simulink model "verify_com_acceleration_computation"  (R2015a)
settings: Solver=ode45  StartTime=0.0  StopTime=1.2  RelTol=1e-3
undefined symbols (not defined in the file or in its folder): A_kalman_transverse, A_kalman_vertical, B_kalman_transverse, B_kalman_vertical, C_kalman_transverse, C_kalman_vertical, com_leg_motor, com_torso, Discrete, g, initial_dx_estimate, initial_dy_estimate, initial_dz_estimate, initial_z_estimate, kalman_stance_slip_threshold, lateral_offset, m_leg, m_leg_motor, m_torso, m_total_real, P0_kalman_transverse, P0_kalman_vertical, pelvis_to_imu, R_kalman_accelerometer, R_kalman_foot_slip, R_kalman_foot_stance, sample_time, Time, X, Y, Z
libraries: nesl_utility x121, sm_lib x43, simulink x3, ctrlSharedLib x3
(part 2 of 3)

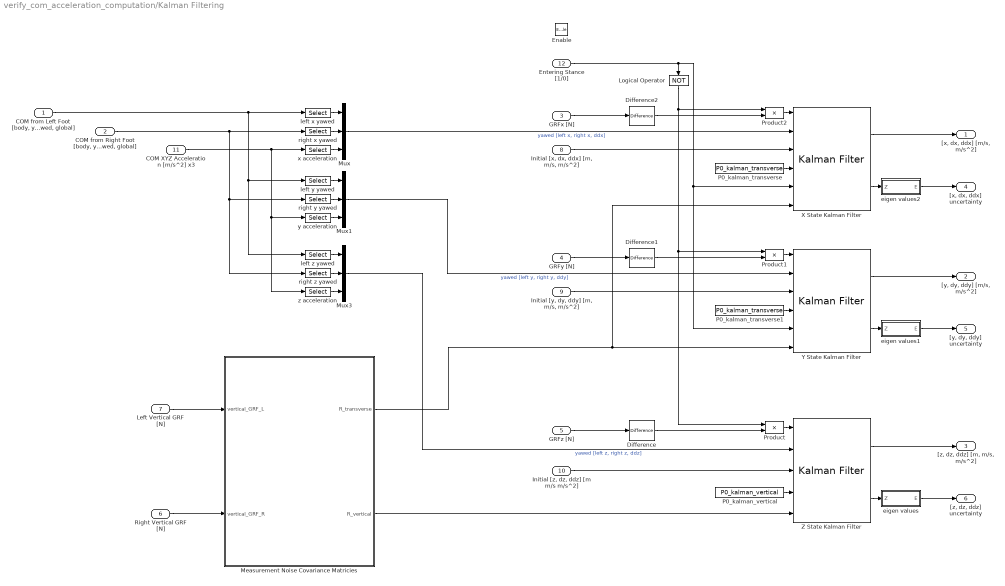
== system verify_com_acceleration_computation/Kalman Filtering ==
  "COM from Left Foot [body, yawed, global]" : Inport  SampleTime=sample_time
  "COM from Right Foot [body, yawed, global]" : Inport  Port=2  SampleTime=sample_time
  GRFx [N] : Inport  Port=3  SampleTime=sample_time
  GRFy [N] : Inport  Port=4  SampleTime=sample_time
  GRFz [N] : Inport  Port=5  SampleTime=sample_time
  Right Vertical GRF [N] : Inport  Port=6  SampleTime=sample_time
  Left Vertical GRF [N] : Inport  Port=7  SampleTime=sample_time
  "Initial [x, dx, ddx] [m, m/s, m/s^2]" : Inport  Port=8  PortDimensions=3  SampleTime=sample_time
  "Initial [y, dy, ddy] [m, m/s, m/s^2]" : Inport  Port=9  PortDimensions=3  SampleTime=sample_time
  "Initial [z, dz, ddz] [m m/s m/s^2]" : Inport  Port=10  PortDimensions=3  SampleTime=sample_time
  COM XYZ Acceleration [m/s^2] x3 : Inport  Port=11  SampleTime=sample_time
  Entering Stance [1/0] : Inport  Port=12  PortDimensions=1  SampleTime=sample_time
  Enable : EnablePort  StatesWhenEnabling=reset
  Difference : simulink/Discrete/Difference  ICPrevInput=0.0  InputProcessing=Inherited  OutMin=[]  OutMax=[]  OutDataType=fixdt(1, 16)  OutScaling=2^-10  DoSatur=off
  Difference1 : simulink/Discrete/Difference  ICPrevInput=0.0  InputProcessing=Inherited  OutMin=[]  OutMax=[]  OutDataType=fixdt(1, 16)  OutScaling=2^-10  DoSatur=off
  Difference2 : simulink/Discrete/Difference  ICPrevInput=0.0  InputProcessing=Inherited  OutMin=[]  OutMax=[]  OutDataType=fixdt(1, 16)  OutScaling=2^-10  DoSatur=off
  Logical Operator : Logic  Operator=NOT  AllPortsSameDT=off  OutDataTypeStr=boolean
  Measurement Noise Covariance Matricies : MATLAB Function  TreatAsAtomicUnit=on
  Mux : Mux  Inputs=3
  Mux1 : Mux  Inputs=3
  Mux3 : Mux  Inputs=3
  P0_kalman_transverse : Constant  Value=P0_kalman_transverse
  P0_kalman_transverse1 : Constant  Value=P0_kalman_transverse
  P0_kalman_vertical : Constant  Value=P0_kalman_vertical
  Product : Product
  Product1 : Product
  Product2 : Product
  X State Kalman Filter : ctrlSharedLib/Kalman Filter  TimeDomain=Discrete-Time  UseCurrentEstimator=on  ModelSource=Individual A, B, C, D matrices  ModelSourceVariable=A_kf  A=A_kalman_transverse  B=B_kalman_transverse  C=C_kalman_transverse  D=0  NumberOfStates=2  NumberOfInputs=1  NumberOfOutputs=2  InitialEstimateSource=Input port  X0=initial_dx_estimate  P0=P0_kalman_transverse  UseK=off  UseGH=on  NumberOfProcessNoiseInputs=1  G=G_kalman_transverse  TimeInvariantG=on  H=0  TimeInvariantH=on  Q=Q_kalman_GRF_difference  TimeInvariantQ=on  R=1  TimeInvariantR=off  N=0  TimeInvariantN=on  AddInputPort=on  AddEnablePort=off  ExternalReset=Rising  OutputEstimatedY=off  OutputP=on  Ts=sample_time
  Y State Kalman Filter : ctrlSharedLib/Kalman Filter  TimeDomain=Discrete-Time  UseCurrentEstimator=on  ModelSource=Individual A, B, C, D matrices  ModelSourceVariable=A_kf  A=A_kalman_transverse  B=B_kalman_transverse  C=C_kalman_transverse  D=0  NumberOfStates=2  NumberOfInputs=1  NumberOfOutputs=2  InitialEstimateSource=Input port  X0=initial_dy_estimate  P0=P0_kalman_transverse  UseK=off  UseGH=on  NumberOfProcessNoiseInputs=1  G=G_kalman_transverse  TimeInvariantG=on  H=0  TimeInvariantH=on  Q=Q_kalman_GRF_difference  TimeInvariantQ=on  R=1  TimeInvariantR=off  N=0  TimeInvariantN=on  AddInputPort=on  AddEnablePort=off  ExternalReset=Rising  OutputEstimatedY=off  OutputP=on  Ts=sample_time
  Z State Kalman Filter : ctrlSharedLib/Kalman Filter  TimeDomain=Discrete-Time  UseCurrentEstimator=on  ModelSource=Individual A, B, C, D matrices  ModelSourceVariable=A_kf  A=A_kalman_vertical  B=B_kalman_vertical  C=C_kalman_vertical  D=0  NumberOfStates=2  NumberOfInputs=1  NumberOfOutputs=2  InitialEstimateSource=Input port  X0=[initial_z_estimate; initial_dz_estimate]  P0=P0_kalman_vertical  UseK=off  UseGH=on  NumberOfProcessNoiseInputs=1  G=G_kalman_vertical  TimeInvariantG=on  H=0  TimeInvariantH=on  Q=Q_kalman_GRF_difference  TimeInvariantQ=on  R=1  TimeInvariantR=off  N=0  TimeInvariantN=on  AddInputPort=on  AddEnablePort=off  OutputEstimatedY=off  OutputP=on  Ts=sample_time
  eigen values : MATLAB Function  TreatAsAtomicUnit=on
  eigen values1 : MATLAB Function  TreatAsAtomicUnit=on
  eigen values2 : MATLAB Function  TreatAsAtomicUnit=on
  left x yawed : Selector  InputPortWidth=9  Indices=[4]
  left y yawed : Selector  InputPortWidth=9  Indices=[5]
  left z yawed : Selector  InputPortWidth=9  Indices=[6]
  right x yawed : Selector  InputPortWidth=9  Indices=[4]
  right y yawed : Selector  InputPortWidth=9  Indices=[5]
  right z yawed : Selector  InputPortWidth=9  Indices=[6]
  x acceleration : Selector  InputPortWidth=3  Indices=[1]
  y acceleration : Selector  InputPortWidth=3  Indices=[2]
  z acceleration : Selector  InputPortWidth=3  Indices=[3]
  "[x, dx, ddx] [m/s, m/s^2]" : Outport
  "[y, dy, ddy] [m/s, m/s^2]" : Outport  Port=2
  "[z, dz, ddz] [m, m/s, m/s^2]" : Outport  Port=3
  "[x, dx, ddx] uncertainty" : Outport  Port=4
  "[y, dy, ddy] uncertainty" : Outport  Port=5
  "[z, dz, ddz] uncertainty" : Outport  Port=6
  wires:
  X State Kalman Filter/1 -> "[x, dx, ddx] [m/s, m/s^2]"/1
  eigen values1/1(E) -> "[y, dy, ddy] uncertainty"/1
  eigen values2/1(E) -> "[x, dx, ddx] uncertainty"/1
  Y State Kalman Filter/1 -> "[y, dy, ddy] [m/s, m/s^2]"/1
  y acceleration/1 -> Mux1/3
  x acceleration/1 -> Mux/3
  z acceleration/1 -> Mux3/3
  COM XYZ Acceleration [m/s^2] x3/1 -> z acceleration/1, y acceleration/1, x acceleration/1
  Z State Kalman Filter/1 -> "[z, dz, ddz] [m, m/s, m/s^2]"/1
  GRFy [N]/1 -> Difference1/1
  Mux3/1 -> Z State Kalman Filter/2  "yawed [left z, right z, ddz]"
  GRFx [N]/1 -> Difference2/1
  Measurement Noise Covariance Matricies/2(R_vertical) -> Z State Kalman Filter/5
  Measurement Noise Covariance Matricies/1(R_transverse) -> X State Kalman Filter/6, Y State Kalman Filter/6
  Mux1/1 -> Y State Kalman Filter/2  "yawed [left y, right y, ddy]"
  Mux/1 -> X State Kalman Filter/2  "yawed [left x, right x, ddx]"
  Right Vertical GRF [N]/1 -> Measurement Noise Covariance Matricies/2(vertical_GRF_R)
  Left Vertical GRF [N]/1 -> Measurement Noise Covariance Matricies/1(vertical_GRF_L)
  "COM from Left Foot [body, yawed, global]"/1 -> left z yawed/1, left y yawed/1, left x yawed/1
  left x yawed/1 -> Mux/1
  "COM from Right Foot [body, yawed, global]"/1 -> right z yawed/1, right y yawed/1, right x yawed/1
  right x yawed/1 -> Mux/2
  left y yawed/1 -> Mux1/1
  right y yawed/1 -> Mux1/2
  left z yawed/1 -> Mux3/1
  right z yawed/1 -> Mux3/2
  P0_kalman_transverse/1 -> X State Kalman Filter/4
  "Initial [x, dx, ddx] [m, m/s, m/s^2]"/1 -> X State Kalman Filter/3
  P0_kalman_transverse1/1 -> Y State Kalman Filter/4
  "Initial [y, dy, ddy] [m, m/s, m/s^2]"/1 -> Y State Kalman Filter/3
  P0_kalman_vertical/1 -> Z State Kalman Filter/4
  "Initial [z, dz, ddz] [m m/s m/s^2]"/1 -> Z State Kalman Filter/3
  X State Kalman Filter/2 -> eigen values2/1(Z)
  Y State Kalman Filter/2 -> eigen values1/1(Z)
  Z State Kalman Filter/2 -> eigen values/1(Z)
  eigen values/1(E) -> "[z, dz, ddz] uncertainty"/1
  Logical Operator/1 -> Product2/1, Product/1, Product1/1
  Difference/1 -> Product/2
  Entering Stance [1/0]/1 -> Y State Kalman Filter/5, X State Kalman Filter/5, Logical Operator/1
  Difference1/1 -> Product1/2
  Difference2/1 -> Product2/2
  Product2/1 -> X State Kalman Filter/1
  Product1/1 -> Y State Kalman Filter/1
  Product/1 -> Z State Kalman Filter/1
  GRFz [N]/1 -> Difference/1

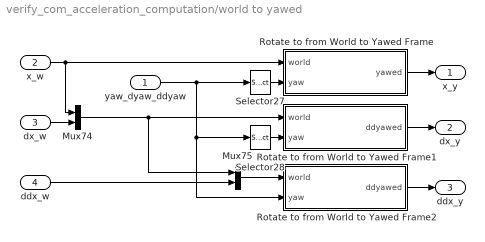
== system verify_com_acceleration_computation/world to yawed ==
  yaw_dyaw_ddyaw : Inport
  x_w : Inport  Port=2
  dx_w : Inport  Port=3
  ddx_w : Inport  Port=4
  Mux74 : Mux  Inputs=2
  Mux75 : Mux  Inputs=2
  Rotate to from World to Yawed Frame : MATLAB Function  TreatAsAtomicUnit=on
  Rotate to from World to Yawed Frame1 : MATLAB Function  TreatAsAtomicUnit=on
  Rotate to from World to Yawed Frame2 : MATLAB Function  TreatAsAtomicUnit=on
  Selector27 : Selector  InputPortWidth=3  Indices=[1]
  Selector28 : Selector  InputPortWidth=3  Indices=[1 2]
  x_y : Outport
  dx_y : Outport  Port=2
  ddx_y : Outport  Port=3
  wires:
  Rotate to from World to Yawed Frame2/1(ddyawed) -> ddx_y/1
  x_w/1 -> Mux74/1, Rotate to from World to Yawed Frame/1(world)
  ddx_w/1 -> Mux75/2
  Mux74/1 -> Mux75/1, Rotate to from World to Yawed Frame1/1(world)
  Mux75/1 -> Rotate to from World to Yawed Frame2/1(world)
  Rotate to from World to Yawed Frame/1(yawed) -> x_y/1
  dx_w/1 -> Mux74/2
  Selector28/1 -> Rotate to from World to Yawed Frame1/2(yaw)
  Rotate to from World to Yawed Frame1/1(ddyawed) -> dx_y/1
  Selector27/1 -> Rotate to from World to Yawed Frame/2(yaw)
  yaw_dyaw_ddyaw/1 -> Selector27/1, Selector28/1, Rotate to from World to Yawed Frame2/2(yaw)

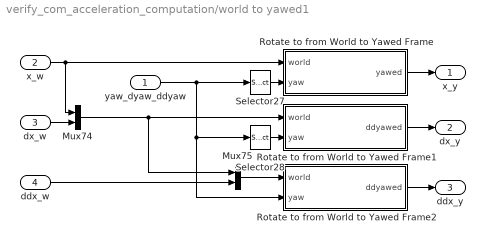
== system verify_com_acceleration_computation/world to yawed1 ==
  yaw_dyaw_ddyaw : Inport
  x_w : Inport  Port=2
  dx_w : Inport  Port=3
  ddx_w : Inport  Port=4
  Mux74 : Mux  Inputs=2
  Mux75 : Mux  Inputs=2
  Rotate to from World to Yawed Frame : MATLAB Function  TreatAsAtomicUnit=on
  Rotate to from World to Yawed Frame1 : MATLAB Function  TreatAsAtomicUnit=on
  Rotate to from World to Yawed Frame2 : MATLAB Function  TreatAsAtomicUnit=on
  Selector27 : Selector  InputPortWidth=3  Indices=[1]
  Selector28 : Selector  InputPortWidth=3  Indices=[1 2]
  x_y : Outport
  dx_y : Outport  Port=2
  ddx_y : Outport  Port=3
  wires:
  Rotate to from World to Yawed Frame2/1(ddyawed) -> ddx_y/1
  x_w/1 -> Mux74/1, Rotate to from World to Yawed Frame/1(world)
  ddx_w/1 -> Mux75/2
  Mux74/1 -> Mux75/1, Rotate to from World to Yawed Frame1/1(world)
  Mux75/1 -> Rotate to from World to Yawed Frame2/1(world)
  Rotate to from World to Yawed Frame/1(yawed) -> x_y/1
  dx_w/1 -> Mux74/2
  Selector28/1 -> Rotate to from World to Yawed Frame1/2(yaw)
  Rotate to from World to Yawed Frame1/1(ddyawed) -> dx_y/1
  Selector27/1 -> Rotate to from World to Yawed Frame/2(yaw)
  yaw_dyaw_ddyaw/1 -> Selector27/1, Selector28/1, Rotate to from World to Yawed Frame2/2(yaw)

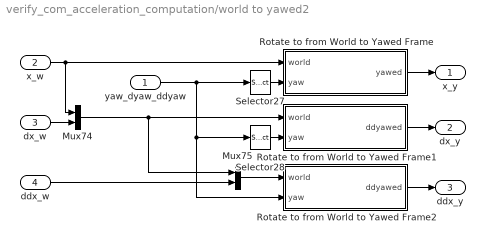
== system verify_com_acceleration_computation/world to yawed2 ==
  yaw_dyaw_ddyaw : Inport
  x_w : Inport  Port=2
  dx_w : Inport  Port=3
  ddx_w : Inport  Port=4
  Mux74 : Mux  Inputs=2
  Mux75 : Mux  Inputs=2
  Rotate to from World to Yawed Frame : MATLAB Function  TreatAsAtomicUnit=on
  Rotate to from World to Yawed Frame1 : MATLAB Function  TreatAsAtomicUnit=on
  Rotate to from World to Yawed Frame2 : MATLAB Function  TreatAsAtomicUnit=on
  Selector27 : Selector  InputPortWidth=3  Indices=[1]
  Selector28 : Selector  InputPortWidth=3  Indices=[1 2]
  x_y : Outport
  dx_y : Outport  Port=2
  ddx_y : Outport  Port=3
  wires:
  Rotate to from World to Yawed Frame2/1(ddyawed) -> ddx_y/1
  x_w/1 -> Mux74/1, Rotate to from World to Yawed Frame/1(world)
  ddx_w/1 -> Mux75/2
  Mux74/1 -> Mux75/1, Rotate to from World to Yawed Frame1/1(world)
  Mux75/1 -> Rotate to from World to Yawed Frame2/1(world)
  Rotate to from World to Yawed Frame/1(yawed) -> x_y/1
  dx_w/1 -> Mux74/2
  Selector28/1 -> Rotate to from World to Yawed Frame1/2(yaw)
  Rotate to from World to Yawed Frame1/1(ddyawed) -> dx_y/1
  Selector27/1 -> Rotate to from World to Yawed Frame/2(yaw)
  yaw_dyaw_ddyaw/1 -> Selector27/1, Selector28/1, Rotate to from World to Yawed Frame2/2(yaw)

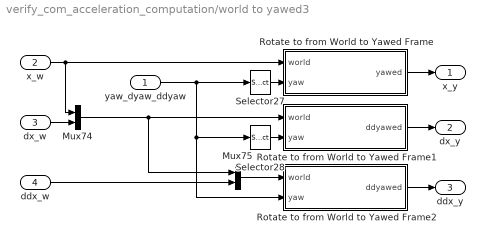
== system verify_com_acceleration_computation/world to yawed3 ==
  yaw_dyaw_ddyaw : Inport
  x_w : Inport  Port=2
  dx_w : Inport  Port=3
  ddx_w : Inport  Port=4
  Mux74 : Mux  Inputs=2
  Mux75 : Mux  Inputs=2
  Rotate to from World to Yawed Frame : MATLAB Function  TreatAsAtomicUnit=on
  Rotate to from World to Yawed Frame1 : MATLAB Function  TreatAsAtomicUnit=on
  Rotate to from World to Yawed Frame2 : MATLAB Function  TreatAsAtomicUnit=on
  Selector27 : Selector  InputPortWidth=3  Indices=[1]
  Selector28 : Selector  InputPortWidth=3  Indices=[1 2]
  x_y : Outport
  dx_y : Outport  Port=2
  ddx_y : Outport  Port=3
  wires:
  Rotate to from World to Yawed Frame2/1(ddyawed) -> ddx_y/1
  x_w/1 -> Mux74/1, Rotate to from World to Yawed Frame/1(world)
  ddx_w/1 -> Mux75/2
  Mux74/1 -> Mux75/1, Rotate to from World to Yawed Frame1/1(world)
  Mux75/1 -> Rotate to from World to Yawed Frame2/1(world)
  Rotate to from World to Yawed Frame/1(yawed) -> x_y/1
  dx_w/1 -> Mux74/2
  Selector28/1 -> Rotate to from World to Yawed Frame1/2(yaw)
  Rotate to from World to Yawed Frame1/1(ddyawed) -> dx_y/1
  Selector27/1 -> Rotate to from World to Yawed Frame/2(yaw)
  yaw_dyaw_ddyaw/1 -> Selector27/1, Selector28/1, Rotate to from World to Yawed Frame2/2(yaw)

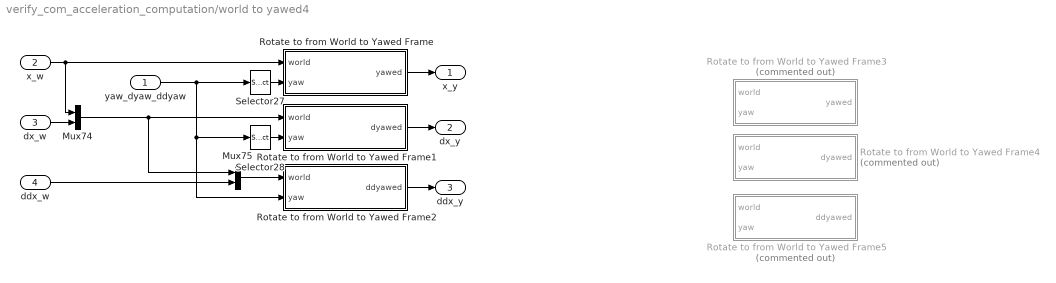
== system verify_com_acceleration_computation/world to yawed4 ==
  yaw_dyaw_ddyaw : Inport
  x_w : Inport  Port=2
  dx_w : Inport  Port=3
  ddx_w : Inport  Port=4
  Mux74 : Mux  Inputs=2
  Mux75 : Mux  Inputs=2
  Rotate to from World to Yawed Frame : MATLAB Function  TreatAsAtomicUnit=on
  Rotate to from World to Yawed Frame1 : MATLAB Function  TreatAsAtomicUnit=on
  Rotate to from World to Yawed Frame2 : MATLAB Function  TreatAsAtomicUnit=on
  Rotate to from World to Yawed Frame3 : MATLAB Function  Commented=on  TreatAsAtomicUnit=on
  Rotate to from World to Yawed Frame4 : MATLAB Function  Commented=on  TreatAsAtomicUnit=on
  Rotate to from World to Yawed Frame5 : MATLAB Function  Commented=on  TreatAsAtomicUnit=on
  Selector27 : Selector  InputPortWidth=3  Indices=[1]
  Selector28 : Selector  InputPortWidth=3  Indices=[1 2]
  x_y : Outport
  dx_y : Outport  Port=2
  ddx_y : Outport  Port=3
  wires:
  yaw_dyaw_ddyaw/1 -> Rotate to from World to Yawed Frame2/2(yaw), Selector28/1, Selector27/1
  Selector27/1 -> Rotate to from World to Yawed Frame/2(yaw)
  Rotate to from World to Yawed Frame1/1(dyawed) -> dx_y/1
  Selector28/1 -> Rotate to from World to Yawed Frame1/2(yaw)
  dx_w/1 -> Mux74/2
  Rotate to from World to Yawed Frame/1(yawed) -> x_y/1
  Mux75/1 -> Rotate to from World to Yawed Frame2/1(world)
  Mux74/1 -> Rotate to from World to Yawed Frame1/1(world), Mux75/1
  ddx_w/1 -> Mux75/2
  x_w/1 -> Rotate to from World to Yawed Frame/1(world), Mux74/1
  Rotate to from World to Yawed Frame2/1(ddyawed) -> ddx_y/1

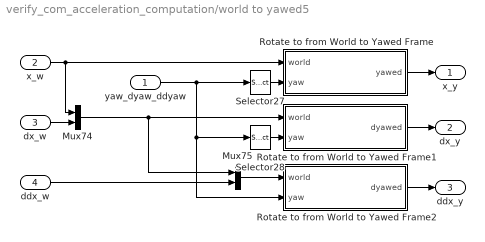
== system verify_com_acceleration_computation/world to yawed5 ==
  yaw_dyaw_ddyaw : Inport
  x_w : Inport  Port=2
  dx_w : Inport  Port=3
  ddx_w : Inport  Port=4
  Mux74 : Mux  Inputs=2
  Mux75 : Mux  Inputs=2
  Rotate to from World to Yawed Frame : MATLAB Function  TreatAsAtomicUnit=on
  Rotate to from World to Yawed Frame1 : MATLAB Function  TreatAsAtomicUnit=on
  Rotate to from World to Yawed Frame2 : MATLAB Function  TreatAsAtomicUnit=on
  Selector27 : Selector  InputPortWidth=3  Indices=[1]
  Selector28 : Selector  InputPortWidth=3  Indices=[1 2]
  x_y : Outport
  dx_y : Outport  Port=2
  ddx_y : Outport  Port=3
  wires:
  Rotate to from World to Yawed Frame2/1(dyawed) -> ddx_y/1
  x_w/1 -> Mux74/1, Rotate to from World to Yawed Frame/1(world)
  ddx_w/1 -> Mux75/2
  Mux74/1 -> Mux75/1, Rotate to from World to Yawed Frame1/1(world)
  Mux75/1 -> Rotate to from World to Yawed Frame2/1(world)
  Rotate to from World to Yawed Frame/1(yawed) -> x_y/1
  dx_w/1 -> Mux74/2
  Selector28/1 -> Rotate to from World to Yawed Frame1/2(yaw)
  Rotate to from World to Yawed Frame1/1(dyawed) -> dx_y/1
  Selector27/1 -> Rotate to from World to Yawed Frame/2(yaw)
  yaw_dyaw_ddyaw/1 -> Selector27/1, Selector28/1, Rotate to from World to Yawed Frame2/2(yaw)

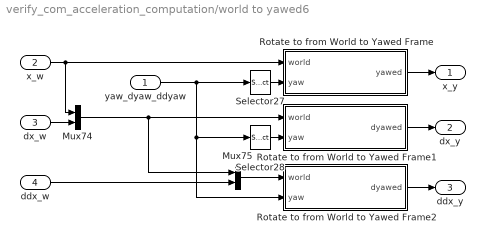
== system verify_com_acceleration_computation/world to yawed6 ==
  yaw_dyaw_ddyaw : Inport
  x_w : Inport  Port=2
  dx_w : Inport  Port=3
  ddx_w : Inport  Port=4
  Mux74 : Mux  Inputs=2
  Mux75 : Mux  Inputs=2
  Rotate to from World to Yawed Frame : MATLAB Function  TreatAsAtomicUnit=on
  Rotate to from World to Yawed Frame1 : MATLAB Function  TreatAsAtomicUnit=on
  Rotate to from World to Yawed Frame2 : MATLAB Function  TreatAsAtomicUnit=on
  Selector27 : Selector  InputPortWidth=3  Indices=[1]
  Selector28 : Selector  InputPortWidth=3  Indices=[1 2]
  x_y : Outport
  dx_y : Outport  Port=2
  ddx_y : Outport  Port=3
  wires:
  yaw_dyaw_ddyaw/1 -> Rotate to from World to Yawed Frame2/2(yaw), Selector28/1, Selector27/1
  Selector27/1 -> Rotate to from World to Yawed Frame/2(yaw)
  Rotate to from World to Yawed Frame1/1(dyawed) -> dx_y/1
  Selector28/1 -> Rotate to from World to Yawed Frame1/2(yaw)
  dx_w/1 -> Mux74/2
  Rotate to from World to Yawed Frame/1(yawed) -> x_y/1
  Mux75/1 -> Rotate to from World to Yawed Frame2/1(world)
  Mux74/1 -> Rotate to from World to Yawed Frame1/1(world), Mux75/1
  ddx_w/1 -> Mux75/2
  x_w/1 -> Rotate to from World to Yawed Frame/1(world), Mux74/1
  Rotate to from World to Yawed Frame2/1(dyawed) -> ddx_y/1

== matlab function verify_com_acceleration_computation/Compute COM Translational Acceleration (IMU uses non-rotating measurement frame) ==
  data: com_acceleration_world output; torso_angular_accelerations input; imu_translational_accelerations_body input; torso_roll input; torso_pitch input; torso_yaw input; com_position_world input; com_velocity_world input; hip_roll_accelerations input; right_hip_roll input; left_hip_roll input; pelvis_to_imu parameter; com_torso parameter; com_leg_motor parameter; m_leg_motor parameter; m_leg parameter; m_torso parameter; torso_com_acceleration_world output; pelvis_acceleration_world output; right_hip_acceleration_world output; left_hip_acceleration_world output; com_acceleration_yawed output
function [com_acceleration_world, torso_com_acceleration_world, pelvis_acceleration_world, right_hip_acceleration_world, left_hip_acceleration_world, com_acceleration_yawed] ...
          = compute_com_acceleration(torso_angular_accelerations, imu_translational_accelerations_body, torso_roll, torso_pitch, torso_yaw, ...
          com_position_world, com_velocity_world, ...
          hip_roll_accelerations, right_hip_roll, left_hip_roll, pelvis_to_imu, com_torso, com_leg_motor, m_leg_motor, m_leg, m_torso)

    % Body frame to Yawed frame rotations  
    R_body_to_yawed = R_pitch(torso_pitch(1))*R_roll(torso_roll(1));
    dR_body_to_yawed = dR_pitch(torso_pitch(1),torso_pitch(2))*R_roll(torso_roll(1)) + R_pitch(torso_pitch(1))*dR_roll(torso_roll(1),torso_roll(2));
    ddR_body_to_yawed = ddR_pitch(torso_pitch(1),torso_pitch(2),torso_angular_accelerations(2))*R_roll(torso_roll(1)) ...
                        + R_pitch(torso_pitch(1))*ddR_roll(torso_roll(1),torso_roll(2),torso_angular_accelerations(1)) ... 
                        + 2*dR_pitch(torso_pitch(1),torso_pitch(2))*dR_roll(torso_roll(1),torso_roll(2));
    % Yawed frame to World frame rotations  
    R_yawed_to_world = R_yaw(torso_yaw(1));
    dR_yawed_to_world = dR_yaw(torso_yaw(1),torso_yaw(2));
    ddR_yawed_to_world = ddR_yaw(torso_yaw(1),torso_yaw(2),torso_angular_accelerations(3));
    % Compute translational acceleration of torso COM
    R_position_body_to_world = R_yawed_to_world*R_body_to_yawed;
    R_velocity_body_to_world = dR_yawed_to_world*R_body_to_yawed + R_yawed_to_world*dR_body_to_yawed;
    R_acceleration_body_to_world = ddR_yawed_to_world*R_body_to_yawed + 2*dR_yawed_to_world*dR_body_to_yawed + R_yawed_to_world*ddR_body_to_yawed;
    imu_to_torso_com_acceleration_world = R_acceleration_body_to_world*(com_torso - pelvis_to_imu)';
    imu_acceleration_world = R_yawed_to_world*R_body_to_yawed*imu_translational_accelerations_body;
    torso_com_acceleration_world = imu_acceleration_world + imu_to_torso_com_acceleration_world;
    % Compute accelerations of hip COMs
    R_right_hip_to_body =     R_roll(-pi/2+right_hip_roll(1));
    dR_right_hip_to_body =   dR_roll(-pi/2+right_hip_roll(1), right_hip_roll(2));
    ddR_right_hip_to_body = ddR_roll(-pi/2+right_hip_roll(1), right_hip_roll(2), hip_roll_accelerations(1));
    R_left_hip_to_body =     R_roll(pi/2-left_hip_roll(1));
    dR_left_hip_to_body =   dR_roll(pi/2-left_hip_roll(1), -left_hip_roll(2));
    ddR_left_hip_to_body = ddR_roll(pi/2-left_hip_roll(1), -left_hip_roll(2), -hip_roll_accelerations(2));
    imu_to_pelvis_com_acceleration_world = R_acceleration_body_to_world*(-pelvis_to_imu)';  
    pelvis_acceleration_world = imu_acceleration_world + imu_to_pelvis_com_acceleration_world;
    left_hip_acceleration_world = pelvis_acceleration_world + (R_acceleration_body_to_world*R_left_hip_to_body + 2*R_velocity_body_to_world*dR_left_hip_to_body + R_position_body_to_world*ddR_left_hip_to_body)*com_leg_motor';
    right_hip_acceleration_world = pelvis_acceleration_world + (R_acceleration_body_to_world*R_right_hip_to_body + 2*R_velocity_body_to_world*dR_right_hip_to_body + R_position_body_to_world*ddR_right_hip_to_body)*(com_leg_motor.*[1,-1,1])';
    % Compute total system COM acceleration
    m_hip = m_leg+m_leg_motor;
    m_total = 2*m_hip + m_torso;
    com_acceleration_world = (m_torso*torso_com_acceleration_world + m_hip*(left_hip_acceleration_world + right_hip_acceleration_world))/m_total;
    com_acceleration_yawed = ddR_yawed_to_world'*com_position_world + 2*dR_yawed_to_world'*com_velocity_world + R_yawed_to_world'*com_acceleration_world;
    %com_acceleration_yawed(3) = com_acceleration_yawed(3) - g;
end

function R_yp = R_pitch(theta) % map from pitched to yawed
  R_yp = [cos(theta), 0, sin(theta); ...
          0, 1, 0; ...
          -sin(theta), 0, cos(theta)];
end
function dR_yp = dR_pitch(theta,dtheta)
  dR_yp = dtheta*[-sin(theta), 0, cos(theta); ...
                  0, 0, 0; ... 
                  -cos(theta), 0, -sin(theta)];
end
function ddR_yp = ddR_pitch(theta,dtheta,ddtheta)
  ddR_yp = ddtheta*[-sin(theta), 0, cos(theta); ...
                    0, 0, 0; ... 
                    -cos(theta), 0, -sin(theta)] ...
           + dtheta^2*[-cos(theta), 0, -sin(theta); ...
                     0, 0, 0; ...
                     sin(theta), 0, -cos(theta)];
end
function R_pr = R_roll(phi) % map from rolled to pitched
  R_pr = [1, 0, 0; ...
          0, cos(phi), -sin(phi); ...
          0, sin(phi), cos(phi)]; 
end
function dR_pr = dR_roll(phi,dphi)
  dR_pr = dphi*[0, 0, 0; ...
                0, -sin(phi), -cos(phi); ...
                0, cos(phi), -sin(phi)];
end
function ddR_pr = ddR_roll(phi, dphi, ddphi)
  ddR_pr = ddphi*[0, 0, 0; ...
                  0, -sin(phi), -cos(phi); ...
                  0, cos(phi), -sin(phi)] ...
           + dphi^2*[0, 0, 0; ...
                   0, -cos(phi), sin(phi);...
                   0, -sin(phi), -cos(phi)];
end
function R_gy = R_yaw(psi) % map yawed frame to global
  R_gy = [cos(psi), -sin(psi), 0; sin(psi), cos(psi), 0; 0 0 1]; 
end
function dR_gy = dR_yaw(psi,dpsi)
  dR_gy = dpsi*[-sin(psi), -cos(psi), 0; cos(psi), -sin(psi), 0; 0 0 0];
end
function ddR_gy = ddR_yaw(psi,dpsi,ddpsi)
  ddR_gy = ddpsi*[-sin(psi), -cos(psi), 0; cos(psi), -sin(psi), 0; 0 0 0] ...
           + dpsi^2*[-cos(psi), sin(psi), 0; -sin(psi), -cos(psi), 0; 0 0 0];
end

== matlab function verify_com_acceleration_computation/Compute COM Translational Acceleration (IMU uses rotating measurement frame)1 ==
  data: com_acceleration_yawed output; torso_angular_accelerations input; imu_translational_positions_body input; imu_translational_velocities_body input; imu_translational_accelerations_body input; torso_roll input; torso_pitch input; hip_roll_accelerations input; right_hip_roll input; left_hip_roll input; pelvis_to_imu parameter; com_torso parameter; com_leg_motor parameter; g parameter; m_leg_motor parameter; m_leg parameter; m_torso parameter; torso_com_acceleration_world output; torso_com_relative_acceleration_world output; torso_com_relative_velocity_world output; imu_to_torso_com_world output; imu_acceleration_world output; imu_velocity_world output; right_hip_acceleration_world output; left_hip_acceleration_world output
function [com_acceleration_yawed,torso_com_acceleration_world,torso_com_relative_acceleration_world,...
          torso_com_relative_velocity_world,imu_to_torso_com_world,imu_acceleration_world,...
          imu_velocity_world, right_hip_acceleration_world, left_hip_acceleration_world] = compute_com_acceleration(torso_angular_accelerations, imu_translational_positions_body, imu_translational_velocities_body, imu_translational_accelerations_body, torso_roll, torso_pitch, hip_roll_accelerations, right_hip_roll, left_hip_roll, pelvis_to_imu, com_torso, com_leg_motor, g, m_leg_motor, m_leg, m_torso)

    % Body frame to Yawed world frame rotations  
    R_body_to_yawed = R_roll(torso_roll(1))*R_pitch(torso_pitch(1));
    dR_body_to_yawed = dR_roll(torso_roll(1),torso_roll(2))*R_pitch(torso_pitch(1)) + R_roll(torso_roll(1))*dR_pitch(torso_pitch(1),torso_pitch(2)); 
    ddR_body_to_yawed = ddR_roll(torso_roll(1),torso_roll(2),torso_angular_accelerations(1))*R_pitch(torso_pitch(1)) ...
                        + R_roll(torso_roll(1))*ddR_pitch(torso_pitch(1),torso_pitch(2),torso_angular_accelerations(2)) ... 
                        + 2*dR_roll(torso_roll(1),torso_roll(2))*dR_pitch(torso_pitch(1),torso_pitch(2)); 
                           
    % Compute translational acceleration of torso COM    
    imu_to_torso_com_world = R_body_to_yawed*(com_torso - pelvis_to_imu)';
    torso_com_relative_velocity_world = dR_body_to_yawed*(com_torso - pelvis_to_imu)';
    torso_com_relative_acceleration_world = ddR_body_to_yawed*(com_torso - pelvis_to_imu)';
    imu_velocity_world = dR_body_to_yawed*imu_translational_positions_body + R_body_to_yawed*imu_translational_velocities_body;
    imu_acceleration_world = ddR_body_to_yawed*imu_translational_positions_body ...
                             + 2*dR_body_to_yawed*imu_translational_velocities_body ...
                             + R_body_to_yawed*imu_translational_accelerations_body;
    torso_com_acceleration_world = imu_acceleration_world + torso_com_relative_acceleration_world;
    
    % Compute accelerations of hip COMs
    R_right_hip_to_body =     R_roll(-pi/2+right_hip_roll(1));
    dR_right_hip_to_body =   dR_roll(-pi/2+right_hip_roll(1), right_hip_roll(2));
    ddR_right_hip_to_body = ddR_roll(-pi/2+right_hip_roll(1), right_hip_roll(2), hip_roll_accelerations(1));
    R_left_hip_to_body =     R_roll(pi/2-left_hip_roll(1));
    dR_left_hip_to_body =   dR_roll(pi/2-left_hip_roll(1), -left_hip_roll(2));
    ddR_left_hip_to_body = ddR_roll(pi/2-left_hip_roll(1), -left_hip_roll(2), -hip_roll_accelerations(2));
    
    pelvis_relative_acceleration_world = ddR_body_to_yawed*(-pelvis_to_imu)';
    pelvis_acceleration_world = imu_acceleration_world + pelvis_relative_acceleration_world;    
    
    left_hip_acceleration_world = pelvis_acceleration_world + (ddR_body_to_yawed*R_left_hip_to_body + 2*(dR_body_to_yawed*dR_left_hip_to_body) + R_body_to_yawed*ddR_left_hip_to_body)*com_leg_motor';
    right_hip_acceleration_world = pelvis_acceleration_world + (ddR_body_to_yawed*R_right_hip_to_body + 2*(dR_body_to_yawed*dR_right_hip_to_body) + R_body_to_yawed*ddR_right_hip_to_body)*(com_leg_motor.*[1,-1,1])';
    
    % Compute total system COM acceleration
    m_hip = m_leg+m_leg_motor;
    m_total = 2*m_hip + m_torso;
    com_acceleration_yawed = (m_torso*torso_com_acceleration_world + m_hip*(left_hip_acceleration_world + right_hip_acceleration_world))/m_total;
     
    
    %com_acceleration_yawed(3) = com_acceleration_yawed(3) - g;
    
end

function R_yp = R_pitch(theta) % map from pitched to yawed
  R_yp = [cos(theta), 0, sin(theta); ...
          0, 1, 0; ...
          -sin(theta), 0, cos(theta)];
end
function dR_yp = dR_pitch(theta,dtheta)
  dR_yp = dtheta*[-sin(theta), 0, cos(theta); ...
                  0, 0, 0; ... 
                  -cos(theta), 0, -sin(theta)];
end
function ddR_yp = ddR_pitch(theta,dtheta,ddtheta)
  ddR_yp = ddtheta*[-sin(theta), 0, cos(theta); ...
                    0, 0, 0; ... 
                    -cos(theta), 0, -sin(theta)] ...
           + dtheta^2*[-cos(theta), 0, -sin(theta); ...
                     0, 0, 0; ...
                     sin(theta), 0, -cos(theta)];
end
function R_pr = R_roll(phi) % map from rolled to pitched
  R_pr = [1, 0, 0; ...
          0, cos(phi), -sin(phi); ...
          0, sin(phi), cos(phi)]; 
end
function dR_pr = dR_roll(phi,dphi)
  dR_pr = dphi*[0, 0, 0; ...
                0, -sin(phi), -cos(phi); ...
                0, cos(phi), -sin(phi)];
end
function ddR_pr = ddR_roll(phi, dphi, ddphi)
  ddR_pr = ddphi*[0, 0, 0; ...
                  0, -sin(phi), -cos(phi); ...
                  0, cos(phi), -sin(phi)] ...
           + dphi^2*[0, 0, 0; ...
                   0, -cos(phi), sin(phi);...
                   0, -sin(phi), -cos(phi)];
end

== matlab function verify_com_acceleration_computation/world to yawed/Rotate to from World to Yawed Frame ==
  data: world input; yawed output; yaw input
function yawed  = WorldToYawed(world, yaw)
    yawed = R_yaw(yaw)'*world;
end

function R_gy = R_yaw(psi) % map yawed frame to global
  R_gy = [cos(psi), -sin(psi), 0; sin(psi), cos(psi), 0; 0 0 1]; 
end

== matlab function verify_com_acceleration_computation/world to yawed/Rotate to from World to Yawed Frame1 ==
  data: world input; ddyawed output; yaw input
function ddyawed  = WorldToYawed(world, yaw)
    ddyawed = dR_yaw(yaw(1),yaw(2))'*world(1:3) + R_yaw(yaw(1))'*world(4:6);
end
function R_gy = R_yaw(psi) % map yawed frame to global
  R_gy = [cos(psi), -sin(psi), 0; sin(psi), cos(psi), 0; 0 0 1]; 
end
function dR_gy = dR_yaw(psi,dpsi)
  dR_gy = dpsi*[-sin(psi), -cos(psi), 0; cos(psi), -sin(psi), 0; 0 0 0];
end

== matlab function verify_com_acceleration_computation/world to yawed/Rotate to from World to Yawed Frame2 ==
  data: world input; ddyawed output; yaw input
function ddyawed  = WorldToYawed(world, yaw)
    ddyawed = ddR_yaw(yaw(1),yaw(2),yaw(3))'*world(1:3) + 2*dR_yaw(yaw(1),yaw(2))'*world(4:6) + R_yaw(yaw(1))'*world(7:9);
end
function R_gy = R_yaw(psi) % map yawed frame to global
  R_gy = [cos(psi), -sin(psi), 0; sin(psi), cos(psi), 0; 0 0 1]; 
end
function dR_gy = dR_yaw(psi,dpsi)
  dR_gy = dpsi*[-sin(psi), -cos(psi), 0; cos(psi), -sin(psi), 0; 0 0 0];
end
function ddR_gy = ddR_yaw(psi,dpsi,ddpsi)
  ddR_gy = ddpsi*[-sin(psi), -cos(psi), 0; cos(psi), -sin(psi), 0; 0 0 0] ...
           + dpsi^2*[-cos(psi), sin(psi), 0; -sin(psi), -cos(psi), 0; 0 0 0];
end

== matlab function verify_com_acceleration_computation/Rotate to from World to Yawed Frame3 ==
  data: world input; yawed output; yaw input
function yawed  = WorldToYawed(world, yaw)
    yawed = R_yaw(yaw)'*world;
end

function R_gy = R_yaw(psi) % map yawed frame to global
  R_gy = [cos(psi), -sin(psi), 0; sin(psi), cos(psi), 0; 0 0 1]; 
end

== matlab function verify_com_acceleration_computation/Rotation To Euler Angles ==
  data: R input; roll output; pitch output; yaw output
function  [roll, pitch, yaw] = rotation_to_euler(R)  
    
    yaw = atan2( R(2,1), R(1,1));
    pitch  = atan2(-R(3,1), sqrt(R(3,2)^2+R(3,3)^2));
    roll   = atan2( R(3,2), R(3,3));

    
%     yaw = atan2(-R(1,2), R(1,1));
%     pitch = atan2(R(1,3), sqrt(R(2,3)^2+R(3,3)^2));
%     roll = atan2(-R(2,3), R(3,3));
    
end

== matlab function verify_com_acceleration_computation/world to yawed1/Rotate to from World to Yawed Frame ==
  data: world input; yawed output; yaw input
function yawed  = WorldToYawed(world, yaw)
    yawed = R_yaw(yaw)'*world;
end

function R_gy = R_yaw(psi) % map yawed frame to global
  R_gy = [cos(psi), -sin(psi), 0; sin(psi), cos(psi), 0; 0 0 1]; 
end

== matlab function verify_com_acceleration_computation/world to yawed1/Rotate to from World to Yawed Frame1 ==
  data: world input; ddyawed output; yaw input
function ddyawed  = WorldToYawed(world, yaw)
    ddyawed = dR_yaw(yaw(1),yaw(2))'*world(1:3) + R_yaw(yaw(1))'*world(4:6);
end
function R_gy = R_yaw(psi) % map yawed frame to global
  R_gy = [cos(psi), -sin(psi), 0; sin(psi), cos(psi), 0; 0 0 1]; 
end
function dR_gy = dR_yaw(psi,dpsi)
  dR_gy = dpsi*[-sin(psi), -cos(psi), 0; cos(psi), -sin(psi), 0; 0 0 0];
end

== matlab function verify_com_acceleration_computation/world to yawed1/Rotate to from World to Yawed Frame2 ==
  data: world input; ddyawed output; yaw input
function ddyawed  = WorldToYawed(world, yaw)
    ddyawed = ddR_yaw(yaw(1),yaw(2),yaw(3))'*world(1:3) + 2*dR_yaw(yaw(1),yaw(2))'*world(4:6) + R_yaw(yaw(1))'*world(7:9);
end
function R_gy = R_yaw(psi) % map yawed frame to global
  R_gy = [cos(psi), -sin(psi), 0; sin(psi), cos(psi), 0; 0 0 1]; 
end
function dR_gy = dR_yaw(psi,dpsi)
  dR_gy = dpsi*[-sin(psi), -cos(psi), 0; cos(psi), -sin(psi), 0; 0 0 0];
end
function ddR_gy = ddR_yaw(psi,dpsi,ddpsi)
  ddR_gy = ddpsi*[-sin(psi), -cos(psi), 0; cos(psi), -sin(psi), 0; 0 0 0] ...
           + dpsi^2*[-cos(psi), sin(psi), 0; -sin(psi), -cos(psi), 0; 0 0 0];
end

== matlab function verify_com_acceleration_computation/Rotate to from World to Yawed Frame1 ==
  data: world input; yawed output; yaw input
function yawed  = WorldToYawed(world, yaw)
    yawed = R_yaw(yaw)'*world;
end

function R_gy = R_yaw(psi) % map yawed frame to global
  R_gy = [cos(psi), -sin(psi), 0; sin(psi), cos(psi), 0; 0 0 1]; 
end

== matlab function verify_com_acceleration_computation/world to yawed2/Rotate to from World to Yawed Frame ==
  data: world input; yawed output; yaw input
function yawed  = WorldToYawed(world, yaw)
    yawed = R_yaw(yaw)'*world;
end

function R_gy = R_yaw(psi) % map yawed frame to global
  R_gy = [cos(psi), -sin(psi), 0; sin(psi), cos(psi), 0; 0 0 1]; 
end

== matlab function verify_com_acceleration_computation/world to yawed2/Rotate to from World to Yawed Frame1 ==
  data: world input; ddyawed output; yaw input
function ddyawed  = WorldToYawed(world, yaw)
    ddyawed = dR_yaw(yaw(1),yaw(2))'*world(1:3) + R_yaw(yaw(1))'*world(4:6);
end
function R_gy = R_yaw(psi) % map yawed frame to global
  R_gy = [cos(psi), -sin(psi), 0; sin(psi), cos(psi), 0; 0 0 1]; 
end
function dR_gy = dR_yaw(psi,dpsi)
  dR_gy = dpsi*[-sin(psi), -cos(psi), 0; cos(psi), -sin(psi), 0; 0 0 0];
end

== matlab function verify_com_acceleration_computation/world to yawed2/Rotate to from World to Yawed Frame2 ==
  data: world input; ddyawed output; yaw input
function ddyawed  = WorldToYawed(world, yaw)
    ddyawed = ddR_yaw(yaw(1),yaw(2),yaw(3))'*world(1:3) + 2*dR_yaw(yaw(1),yaw(2))'*world(4:6) + R_yaw(yaw(1))'*world(7:9);
end
function R_gy = R_yaw(psi) % map yawed frame to global
  R_gy = [cos(psi), -sin(psi), 0; sin(psi), cos(psi), 0; 0 0 1]; 
end
function dR_gy = dR_yaw(psi,dpsi)
  dR_gy = dpsi*[-sin(psi), -cos(psi), 0; cos(psi), -sin(psi), 0; 0 0 0];
end
function ddR_gy = ddR_yaw(psi,dpsi,ddpsi)
  ddR_gy = ddpsi*[-sin(psi), -cos(psi), 0; cos(psi), -sin(psi), 0; 0 0 0] ...
           + dpsi^2*[-cos(psi), sin(psi), 0; -sin(psi), -cos(psi), 0; 0 0 0];
end

== matlab function verify_com_acceleration_computation/Rotate to from World to Yawed Frame2 ==
  data: world input; yawed output; yaw input
function yawed  = WorldToYawed(world, yaw)
    yawed = R_yaw(yaw)'*world;
end

function R_gy = R_yaw(psi) % map yawed frame to global
  R_gy = [cos(psi), -sin(psi), 0; sin(psi), cos(psi), 0; 0 0 1]; 
end

== matlab function verify_com_acceleration_computation/world to yawed3/Rotate to from World to Yawed Frame ==
  data: world input; yawed output; yaw input
function yawed  = WorldToYawed(world, yaw)
    yawed = R_yaw(yaw)'*world;
end

function R_gy = R_yaw(psi) % map yawed frame to global
  R_gy = [cos(psi), -sin(psi), 0; sin(psi), cos(psi), 0; 0 0 1]; 
end

== matlab function verify_com_acceleration_computation/world to yawed3/Rotate to from World to Yawed Frame1 ==
  data: world input; ddyawed output; yaw input
function ddyawed  = WorldToYawed(world, yaw)
    ddyawed = dR_yaw(yaw(1),yaw(2))'*world(1:3) + R_yaw(yaw(1))'*world(4:6);
end
function R_gy = R_yaw(psi) % map yawed frame to global
  R_gy = [cos(psi), -sin(psi), 0; sin(psi), cos(psi), 0; 0 0 1]; 
end
function dR_gy = dR_yaw(psi,dpsi)
  dR_gy = dpsi*[-sin(psi), -cos(psi), 0; cos(psi), -sin(psi), 0; 0 0 0];
end

== matlab function verify_com_acceleration_computation/world to yawed3/Rotate to from World to Yawed Frame2 ==
  data: world input; ddyawed output; yaw input
function ddyawed  = WorldToYawed(world, yaw)
    ddyawed = ddR_yaw(yaw(1),yaw(2),yaw(3))'*world(1:3) + 2*dR_yaw(yaw(1),yaw(2))'*world(4:6) + R_yaw(yaw(1))'*world(7:9);
end
function R_gy = R_yaw(psi) % map yawed frame to global
  R_gy = [cos(psi), -sin(psi), 0; sin(psi), cos(psi), 0; 0 0 1]; 
end
function dR_gy = dR_yaw(psi,dpsi)
  dR_gy = dpsi*[-sin(psi), -cos(psi), 0; cos(psi), -sin(psi), 0; 0 0 0];
end
function ddR_gy = ddR_yaw(psi,dpsi,ddpsi)
  ddR_gy = ddpsi*[-sin(psi), -cos(psi), 0; cos(psi), -sin(psi), 0; 0 0 0] ...
           + dpsi^2*[-cos(psi), sin(psi), 0; -sin(psi), -cos(psi), 0; 0 0 0];
end

== matlab function verify_com_acceleration_computation/world to yawed4/Rotate to from World to Yawed Frame ==
  data: world input; yawed output; yaw input
function yawed  = WorldToYawed(world, yaw)
    yawed = R_yaw(yaw)'*world;
end

function R_gy = R_yaw(psi) % map yawed frame to global
  R_gy = [cos(psi), -sin(psi), 0; sin(psi), cos(psi), 0; 0 0 1]; 
end

== matlab function verify_com_acceleration_computation/world to yawed4/Rotate to from World to Yawed Frame1 ==
  data: world input; dyawed output; yaw input
function dyawed  = WorldToYawed(world, yaw)
    dyawed = R_yaw(yaw(1))'*world(4:6);
end
function R_gy = R_yaw(psi) % map yawed frame to global
  R_gy = [cos(psi), -sin(psi), 0; sin(psi), cos(psi), 0; 0 0 1]; 
end
function dR_gy = dR_yaw(psi,dpsi)
  dR_gy = dpsi*[-sin(psi), -cos(psi), 0; cos(psi), -sin(psi), 0; 0 0 0];
end

== matlab function verify_com_acceleration_computation/world to yawed4/Rotate to from World to Yawed Frame2 ==
  data: world input; ddyawed output; yaw input
function ddyawed  = WorldToYawed(world, yaw)
    ddyawed = R_yaw(yaw(1))'*world(7:9);
end
function R_gy = R_yaw(psi) % map yawed frame to global
  R_gy = [cos(psi), -sin(psi), 0; sin(psi), cos(psi), 0; 0 0 1]; 
end
function dR_gy = dR_yaw(psi,dpsi)
  dR_gy = dpsi*[-sin(psi), -cos(psi), 0; cos(psi), -sin(psi), 0; 0 0 0];
end
function ddR_gy = ddR_yaw(psi,dpsi,ddpsi)
  ddR_gy = ddpsi*[-sin(psi), -cos(psi), 0; cos(psi), -sin(psi), 0; 0 0 0] ...
           + dpsi^2*[-cos(psi), sin(psi), 0; -sin(psi), -cos(psi), 0; 0 0 0];
end

== matlab function verify_com_acceleration_computation/world to yawed5/Rotate to from World to Yawed Frame ==
  data: world input; yawed output; yaw input
function yawed  = WorldToYawed(world, yaw)
    yawed = R_yaw(yaw)'*world;
end

function R_gy = R_yaw(psi) % map yawed frame to global
  R_gy = [cos(psi), -sin(psi), 0; sin(psi), cos(psi), 0; 0 0 1]; 
end

== matlab function verify_com_acceleration_computation/world to yawed5/Rotate to from World to Yawed Frame1 ==
  data: world input; dyawed output; yaw input
function dyawed  = WorldToYawed(world, yaw)
    dyawed = R_yaw(yaw(1))'*world(4:6);
end
function R_gy = R_yaw(psi) % map yawed frame to global
  R_gy = [cos(psi), -sin(psi), 0; sin(psi), cos(psi), 0; 0 0 1]; 
end
function dR_gy = dR_yaw(psi,dpsi)
  dR_gy = dpsi*[-sin(psi), -cos(psi), 0; cos(psi), -sin(psi), 0; 0 0 0];
end

== matlab function verify_com_acceleration_computation/world to yawed5/Rotate to from World to Yawed Frame2 ==
  data: world input; dyawed output; yaw input
function dyawed  = WorldToYawed(world, yaw)
    dyawed = R_yaw(yaw(1))'*world(7:9);
end
function R_gy = R_yaw(psi) % map yawed frame to global
  R_gy = [cos(psi), -sin(psi), 0; sin(psi), cos(psi), 0; 0 0 1]; 
end
function dR_gy = dR_yaw(psi,dpsi)
  dR_gy = dpsi*[-sin(psi), -cos(psi), 0; cos(psi), -sin(psi), 0; 0 0 0];
end
function ddR_gy = ddR_yaw(psi,dpsi,ddpsi)
  ddR_gy = ddpsi*[-sin(psi), -cos(psi), 0; cos(psi), -sin(psi), 0; 0 0 0] ...
           + dpsi^2*[-cos(psi), sin(psi), 0; -sin(psi), -cos(psi), 0; 0 0 0];
end

== matlab function verify_com_acceleration_computation/world to yawed6/Rotate to from World to Yawed Frame ==
  data: world input; yawed output; yaw input
function yawed  = WorldToYawed(world, yaw)
    yawed = R_yaw(yaw)'*world;
end

function R_gy = R_yaw(psi) % map yawed frame to global
  R_gy = [cos(psi), -sin(psi), 0; sin(psi), cos(psi), 0; 0 0 1]; 
end

== matlab function verify_com_acceleration_computation/world to yawed6/Rotate to from World to Yawed Frame1 ==
  data: world input; dyawed output; yaw input
function dyawed  = WorldToYawed(world, yaw)
    dyawed = R_yaw(yaw(1))'*world(4:6);
end
function R_gy = R_yaw(psi) % map yawed frame to global
  R_gy = [cos(psi), -sin(psi), 0; sin(psi), cos(psi), 0; 0 0 1]; 
end
function dR_gy = dR_yaw(psi,dpsi)
  dR_gy = dpsi*[-sin(psi), -cos(psi), 0; cos(psi), -sin(psi), 0; 0 0 0];
end

== matlab function verify_com_acceleration_computation/world to yawed6/Rotate to from World to Yawed Frame2 ==
  data: world input; dyawed output; yaw input
function dyawed  = WorldToYawed(world, yaw)
    dyawed = R_yaw(yaw(1))'*world(7:9);
end
function R_gy = R_yaw(psi) % map yawed frame to global
  R_gy = [cos(psi), -sin(psi), 0; sin(psi), cos(psi), 0; 0 0 1]; 
end
function dR_gy = dR_yaw(psi,dpsi)
  dR_gy = dpsi*[-sin(psi), -cos(psi), 0; cos(psi), -sin(psi), 0; 0 0 0];
end
function ddR_gy = ddR_yaw(psi,dpsi,ddpsi)
  ddR_gy = ddpsi*[-sin(psi), -cos(psi), 0; cos(psi), -sin(psi), 0; 0 0 0] ...
           + dpsi^2*[-cos(psi), sin(psi), 0; -sin(psi), -cos(psi), 0; 0 0 0];
end

== matlab function verify_com_acceleration_computation/world to yawed4/Rotate to from World to Yawed Frame3 ==
  data: world input; yawed output; yaw input
function yawed  = WorldToYawed(world, yaw)
    yawed = R_yaw(yaw)'*world;
end

function R_gy = R_yaw(psi) % map yawed frame to global
  R_gy = [cos(psi), -sin(psi), 0; sin(psi), cos(psi), 0; 0 0 1]; 
end

== matlab function verify_com_acceleration_computation/world to yawed4/Rotate to from World to Yawed Frame4 ==
  data: world input; dyawed output; yaw input
function dyawed  = WorldToYawed(world, yaw)
    dyawed = dR_yaw(yaw(1),yaw(2))'*world(1:3) + R_yaw(yaw(1))'*world(4:6);
end
function R_gy = R_yaw(psi) % map yawed frame to global
  R_gy = [cos(psi), -sin(psi), 0; sin(psi), cos(psi), 0; 0 0 1]; 
end
function dR_gy = dR_yaw(psi,dpsi)
  dR_gy = dpsi*[-sin(psi), -cos(psi), 0; cos(psi), -sin(psi), 0; 0 0 0];
end

== matlab function verify_com_acceleration_computation/world to yawed4/Rotate to from World to Yawed Frame5 ==
  data: world input; ddyawed output; yaw input
function ddyawed  = WorldToYawed(world, yaw)
    ddyawed = ddR_yaw(yaw(1),yaw(2),yaw(3))'*world(1:3) + 2*dR_yaw(yaw(1),yaw(2))'*world(4:6) + R_yaw(yaw(1))'*world(7:9);
end
function R_gy = R_yaw(psi) % map yawed frame to global
  R_gy = [cos(psi), -sin(psi), 0; sin(psi), cos(psi), 0; 0 0 1]; 
end
function dR_gy = dR_yaw(psi,dpsi)
  dR_gy = dpsi*[-sin(psi), -cos(psi), 0; cos(psi), -sin(psi), 0; 0 0 0];
end
function ddR_gy = ddR_yaw(psi,dpsi,ddpsi)
  ddR_gy = ddpsi*[-sin(psi), -cos(psi), 0; cos(psi), -sin(psi), 0; 0 0 0] ...
           + dpsi^2*[-cos(psi), sin(psi), 0; -sin(psi), -cos(psi), 0; 0 0 0];
end

== matlab function verify_com_acceleration_computation/Compute COM Translational Acceleration (IMU uses non-rotating measurement frame) (yawed frame as rotated world frame - non rotating) ==
  data: com_acceleration_yawed output; torso_angular_accelerations input; imu_translational_accelerations_body input; torso_roll input; torso_pitch input; torso_yaw input; hip_roll_accelerations input; right_hip_roll input; left_hip_roll input; pelvis_to_imu parameter; com_torso parameter; com_leg_motor parameter; m_leg_motor parameter; m_leg parameter; m_torso parameter; torso_com_acceleration_yawed output; imu_to_torso_com_acceleration_yawed output; imu_to_torso_com_velocity_yawed output; imu_to_torso_com_position_yawed output; imu_acceleration_yawed output; imu_to_pelvis_acceleration_yawed output; pelvis_acceleration_yawed output; right_hip_acceleration_yawed output; left_hip_acceleration_yawed output
function [com_acceleration_yawed,torso_com_acceleration_yawed,imu_to_torso_com_acceleration_yawed,...
          imu_to_torso_com_velocity_yawed,imu_to_torso_com_position_yawed,imu_acceleration_yawed,...
          imu_to_pelvis_acceleration_yawed, pelvis_acceleration_yawed, right_hip_acceleration_yawed, left_hip_acceleration_yawed] ...
          = compute_com_acceleration(torso_angular_accelerations, imu_translational_accelerations_body, torso_roll, torso_pitch, torso_yaw, ...
          hip_roll_accelerations, right_hip_roll, left_hip_roll, pelvis_to_imu, com_torso, com_leg_motor, m_leg_motor, m_leg, m_torso)

    % Body frame to Yawed frame rotations  
    R_body_to_yawed = R_pitch(torso_pitch(1))*R_roll(torso_roll(1));
    dR_body_to_yawed = dR_pitch(torso_pitch(1),torso_pitch(2))*R_roll(torso_roll(1)) + R_pitch(torso_pitch(1))*dR_roll(torso_roll(1),torso_roll(2));
    ddR_body_to_yawed = ddR_pitch(torso_pitch(1),torso_pitch(2),torso_angular_accelerations(2))*R_roll(torso_roll(1)) ...
                        + R_pitch(torso_pitch(1))*ddR_roll(torso_roll(1),torso_roll(2),torso_angular_accelerations(1)) ... 
                        + 2*dR_pitch(torso_pitch(1),torso_pitch(2))*dR_roll(torso_roll(1),torso_roll(2));
    % Yawed frame to World frame rotations  
    R_yawed_to_world = R_yaw(torso_yaw(1));
    dR_yawed_to_world = dR_yaw(torso_yaw(1),torso_yaw(2));
    ddR_yawed_to_world = ddR_yaw(torso_yaw(1),torso_yaw(2),torso_angular_accelerations(3));
    % Compute translational acceleration of torso COM    
    imu_to_torso_com_position_yawed = R_body_to_yawed*(com_torso - pelvis_to_imu)';
    R_velocity_body_to_yawed = R_yawed_to_world'*(dR_yawed_to_world*R_body_to_yawed + R_yawed_to_world*dR_body_to_yawed);
    imu_to_torso_com_velocity_yawed = R_velocity_body_to_yawed*(com_torso - pelvis_to_imu)';
    R_acceleration_body_to_yawed = R_yawed_to_world'*(ddR_yawed_to_world*R_body_to_yawed + 2*dR_yawed_to_world*dR_body_to_yawed + R_yawed_to_world*ddR_body_to_yawed);
    imu_to_torso_com_acceleration_yawed =  R_acceleration_body_to_yawed*(com_torso - pelvis_to_imu)';
    imu_acceleration_yawed = R_body_to_yawed*imu_translational_accelerations_body;
    torso_com_acceleration_yawed = imu_acceleration_yawed + imu_to_torso_com_acceleration_yawed;
    % Compute accelerations of hip COMs
    R_right_hip_to_body =     R_roll(-pi/2+right_hip_roll(1));
    dR_right_hip_to_body =   dR_roll(-pi/2+right_hip_roll(1), right_hip_roll(2));
    ddR_right_hip_to_body = ddR_roll(-pi/2+right_hip_roll(1), right_hip_roll(2), hip_roll_accelerations(1));
    R_left_hip_to_body =     R_roll(pi/2-left_hip_roll(1));
    dR_left_hip_to_body =   dR_roll(pi/2-left_hip_roll(1), -left_hip_roll(2));
    ddR_left_hip_to_body = ddR_roll(pi/2-left_hip_roll(1), -left_hip_roll(2), -hip_roll_accelerations(2));
    imu_to_pelvis_acceleration_yawed = R_acceleration_body_to_yawed*(-pelvis_to_imu)';
    pelvis_acceleration_yawed = imu_acceleration_yawed + imu_to_pelvis_acceleration_yawed;    
    left_hip_acceleration_yawed = pelvis_acceleration_yawed + (R_acceleration_body_to_yawed*R_left_hip_to_body + 2*R_velocity_body_to_yawed*dR_left_hip_to_body + R_body_to_yawed*ddR_left_hip_to_body)*com_leg_motor';
    right_hip_acceleration_yawed = pelvis_acceleration_yawed + (R_acceleration_body_to_yawed*R_right_hip_to_body + 2*R_velocity_body_to_yawed*dR_right_hip_to_body + R_body_to_yawed*ddR_right_hip_to_body)*(com_leg_motor.*[1,-1,1])';
    % Compute total system COM acceleration
    m_hip = m_leg+m_leg_motor;
    m_total = 2*m_hip + m_torso;
    com_acceleration_yawed = (m_torso*torso_com_acceleration_yawed + m_hip*(left_hip_acceleration_yawed + right_hip_acceleration_yawed))/m_total;
    %com_acceleration_yawed(3) = com_acceleration_yawed(3) - g;
end

function R_yp = R_pitch(theta) % map from pitched to yawed
  R_yp = [cos(theta), 0, sin(theta); ...
          0, 1, 0; ...
          -sin(theta), 0, cos(theta)];
end
function dR_yp = dR_pitch(theta,dtheta)
  dR_yp = dtheta*[-sin(theta), 0, cos(theta); ...
                  0, 0, 0; ... 
                  -cos(theta), 0, -sin(theta)];
end
function ddR_yp = ddR_pitch(theta,dtheta,ddtheta)
  ddR_yp = ddtheta*[-sin(theta), 0, cos(theta); ...
                    0, 0, 0; ... 
                    -cos(theta), 0, -sin(theta)] ...
           + dtheta^2*[-cos(theta), 0, -sin(theta); ...
                     0, 0, 0; ...
                     sin(theta), 0, -cos(theta)];
end
function R_pr = R_roll(phi) % map from rolled to pitched
  R_pr = [1, 0, 0; ...
          0, cos(phi), -sin(phi); ...
          0, sin(phi), cos(phi)]; 
end
function dR_pr = dR_roll(phi,dphi)
  dR_pr = dphi*[0, 0, 0; ...
                0, -sin(phi), -cos(phi); ...
                0, cos(phi), -sin(phi)];
end
function ddR_pr = ddR_roll(phi, dphi, ddphi)
  ddR_pr = ddphi*[0, 0, 0; ...
                  0, -sin(phi), -cos(phi); ...
                  0, cos(phi), -sin(phi)] ...
           + dphi^2*[0, 0, 0; ...
                   0, -cos(phi), sin(phi);...
                   0, -sin(phi), -cos(phi)];
end
function R_gy = R_yaw(psi) % map yawed frame to global
  R_gy = [cos(psi), -sin(psi), 0; sin(psi), cos(psi), 0; 0 0 1]; 
end
function dR_gy = dR_yaw(psi,dpsi)
  dR_gy = dpsi*[-sin(psi), -cos(psi), 0; cos(psi), -sin(psi), 0; 0 0 0];
end
function ddR_gy = ddR_yaw(psi,dpsi,ddpsi)
  ddR_gy = ddpsi*[-sin(psi), -cos(psi), 0; cos(psi), -sin(psi), 0; 0 0 0] ...
           + dpsi^2*[-cos(psi), sin(psi), 0; -sin(psi), -cos(psi), 0; 0 0 0];
end
